simulink model "notcontroledsystem"  (R2018b)
settings: Solver=ode45  StartTime=0.0  StopTime=30  RelTol=1e-3
settings Model: Creator=ASUS  LastModifiedBy=ASUS
settings DataIOCC: LimitDataPoints=on  SaveFormat=Array
settings OptimizationCC: BlockReduction=off  BooleanDataType=off  LifeSpan=inf
settings DebuggingCC: SaveWithParameterizedLinksMsg=none  UnderspecifiedInitializationDetection=Classic  MergeDetectMultiDrivingBlocksExec=none  SignalResolutionControl=TryResolveAllWithWarning  SFUnexpectedBacktrackingDiag=warning  SFNoUnconditionalDefaultTransitionDiag=warning  SFExecutionAtInitializationDiag=none
settings HardwareCC: ProdBitPerPointer=32  ProdBitPerSizeT=32  ProdBitPerPtrDiffT=32  ProdLargestAtomicFloat=None  ProdIntDivRoundTo=Undefined  ProdEndianess=Unspecified  ProdWordSize=32  ProdHWDeviceType=32-bit Generic  TargetUnknown=on
settings ModelReferenceCC: PropagateSignalLabelsOutOfModel=off
settings SFSimCC: SimUseLocalCustomCode=off
settings RTWCC: RTWUseLocalCustomCode=off
settings CodeAppCC: StateflowObjectComments=on
settings GRTTargetCC: TargetLangStandard=C89/C90 (ANSI)  GeneratePreprocessorConditionals=Disable all
settings ConfigComp: CovMetricSettings=dw  CovHtmlReporting=on  CovSaveCumulativeToWorkspaceVar=on  CovSaveSingleToWorkspaceVar=on  CovExternalEMLEnable=off  CovSFcnEnable=off

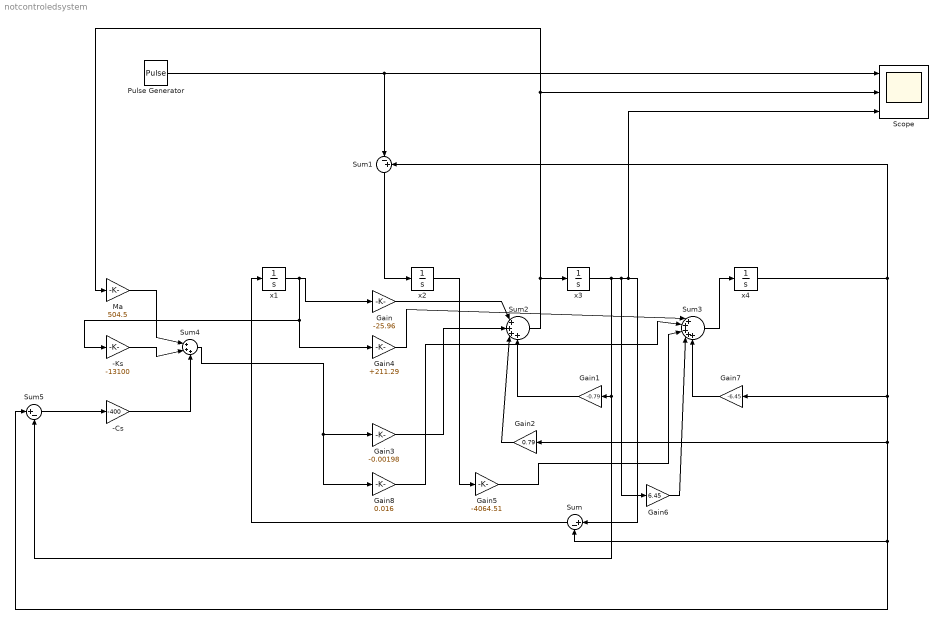
== system notcontroledsystem ==
  "-Cs " : Gain  Gain=-400
  -Ks : Gain  Gain=-13100
  Gain : Gain  Gain=-25.96
  Gain1 : Gain  Gain=-0.79
  Gain2 : Gain  Gain=0.79
  Gain3 : Gain  Gain=-0.00198
  Gain4 : Gain  Gain=+211.29
  Gain5 : Gain  Gain=-4064.51
  Gain6 : Gain  Gain=6.45
  Gain7 : Gain  Gain=-6.45
  Gain8 : Gain  Gain=0.016
  Ma : Gain  Gain=504.5
  Pulse Generator : DiscretePulseGenerator  PulseType=Time based  Period=10  PulseWidth=15
  Scope : Scope  NumInputPorts=3
  Sum : Sum  Inputs=|+-
  Sum1 : Sum  Inputs=|-+
  Sum2 : Sum  Inputs=|++++
  Sum3 : Sum  Inputs=|+++++
  Sum4 : Sum  Inputs=|+++
  Sum5 : Sum  Inputs=|+-
  x{1..4} (4 alike) : Integrator
  wires:
  Sum/1 -> x1/1
  x1/1 -> Gain4/1, -Ks/1, Gain/1
  x2/1 -> Gain5/1
  Sum3/1 -> x4/1
  x4/1 -> Sum5/1, Sum/2, Gain2/1, Gain7/1, Sum1/2
  Gain/1 -> Sum2/1
  Gain3/1 -> Sum2/2
  Gain2/1 -> Sum2/3
  Gain1/1 -> Sum2/4
  Gain4/1 -> Sum3/1
  Gain8/1 -> Sum3/2
  Gain5/1 -> Sum3/3
  Gain6/1 -> Sum3/4
  Gain7/1 -> Sum3/5
  Sum4/1 -> Gain8/1, Gain3/1
  x3/1 -> Sum5/2, Gain1/1, Gain6/1, Scope/3, Sum/1
  Sum1/1 -> x2/1
  Sum2/1 -> x3/1, Ma/1, Scope/2
  Sum5/1 -> "-Cs "/1
  Ma/1 -> Sum4/1
  -Ks/1 -> Sum4/2
  "-Cs "/1 -> Sum4/3
  Pulse Generator/1 -> Scope/1, Sum1/1
